simulink model "advanced_3d_lookup"  (R2023a)
settings: Solver=ode1  StartTime=0  StopTime=400  FixedStep=0.002  RelTol=1e-3  EnableMultiTasking=on
values from neighbouring files (symbols this model uses):
  B = b*L*(K_v)^2 /J_xx    (= 0.042375883612)    [advanced_model_setup.m]    (also in brusselator.m = 2.15; cycle_detection.m = img2; cycle_detection_start.m = img2; demonstrateDetections.m = 2.15)
  beta3d = 0.9    [advanced_model_setup.m]
  cycleGain = 0.1    [advanced_model_setup.m]
  epsilon3d = 1    [advanced_model_setup.m]    (also in gainScheduling.m = evalin('base', 'epsilon3d'))
  f_p = 1.3    [advanced_model_setup.m]    (also in modelCompPlot.m)
  f_r = 0.4    [advanced_model_setup.m]    (also in modelCompPlot.m)
  f_y = 0.175    [advanced_model_setup.m]    (also in modelCompPlot.m)
  g_p = 10.5    [advanced_model_setup.m]    (also in modelCompPlot.m)
  g_r = 5.2    [advanced_model_setup.m]    (also in modelCompPlot.m)
  I_xx = 0.0522    [advanced_model_setup.m]    (also in modelCompPlot.m; set_model_params.m; solveSyms3d_2.m = evalin('base', 'I_xx'))
  I_yy = 0.0522    [advanced_model_setup.m]    (also in modelCompPlot.m; set_model_params.m; solveSyms3d_2.m = evalin('base', 'I_yy'))
  I_zz = 0.1104    [advanced_model_setup.m]    (also in modelCompPlot.m; set_model_params.m; solveSyms3d_2.m = evalin('base', 'I_zz'))
  J = (J_yy - J_zz)/J_xx    (= -1)    [advanced_model_setup.m]    (also in modelCompPlot.m)
  J_r = J_inertia/J_xx    (= 0.00108695652174)    [advanced_model_setup.m]    (also in modelCompPlot.m; solveSyms3d.m = evalin('base', 'J_r'))
  k3d = 1.65    [advanced_model_setup.m]    (also in gainScheduling.m = evalin('base', 'k3d'))
  K_v = 54.945    [advanced_model_setup.m]    (also in modelCompPlot.m; solveSyms3d.m = evalin('base', 'K_v'))
  kfr_p = 0.4*u2line/x5line    (= 0.285774113641)    [advanced_model_setup.m]    (also in modelCompPlot.m; set_model_params.m)
  kfr_r = 0.4*u1line/x4line    (= 0.285774113641)    [advanced_model_setup.m]    (also in modelCompPlot.m; set_model_params.m)
  kfr_y = 0.4*u3line/x6line    (= 0.0880063173321)    [advanced_model_setup.m]    (also in modelCompPlot.m; set_model_params.m)
  sigma = 0    [modelCompPlot.m]
  u1_T = zeros(x5L, x6L, u10L, u20L)    [lookup_gen_optimal.m]
  u2_T = zeros(x5L, x6L, u10L, u20L)    [lookup_gen_optimal.m]
  u3_T = zeros(x5L, x6L, u10L, u20L)    [lookup_gen_optimal.m]
  u4_T = zeros(x5L, x6L, u10L, u20L)    [lookup_gen_optimal.m]
  V_bias = 12    [advanced_model_setup.m]    (also in modelCompPlot.m; set_model_params.m; solveSyms3d.m = evalin('base', 'V_bias'))
  velMax = 1000    [advanced_model_setup.m]
  wcf = 2 * pi * 20    (= 125.663706144)    [advanced_model_setup.m]    (also in modelCompPlot.m; set_model_params.m)
  x5_range = -45:5:45    [lookup_gen_optimal.m]
  x6_range = -45:5:45    [lookup_gen_optimal.m]
  Y = d*(K_v)^2 /J_zz    (= 0.0032609614876)    [advanced_model_setup.m]    (also in modelCompPlot.m; solveSyms3d.m = evalin('base', 'Y'))
  zetaf = 0.6    [advanced_model_setup.m]    (also in modelCompPlot.m; set_model_params.m)
undefined symbols (not defined in the file or in its folder): u00_range
libraries: simulink_extras x2, dspsrcs4 x1
settings Model: ExtModeTrigDuration=10000  Creator=kille  LastModifiedBy=Jacob
settings SolverCC: PositivePriorityOrder=on  AutoInsertRateTranBlk=on
settings DataIOCC: ReturnWorkspaceOutputs=off
settings OptimizationCC: LifeSpan=inf
settings DebuggingCC: UnconnectedInputMsg=warning  UnconnectedOutputMsg=warning  UnconnectedLineMsg=warning  ArithmeticOperatorsInVariantConditions=warning
settings ModelReferenceCC: EnableRefExpFcnMdlSchedulingChecks=on
settings SFSimCC: SimUseLocalCustomCode=off  CustomCodeUndefinedFunction=UseInterfaceOnly
settings RTWCC: Description=QUARC Win64 Target  SystemTargetFile=quarc_win64.tlc  TemplateMakefile=quarc_default_tmf  RTWUseLocalCustomCode=off
settings CodeAppCC: StateflowObjectComments=on
settings STFCustomTargetCC: TargetPreCompLibLocation=C:\PROGRA~3\QUARC\lib\2016a\win64\release  UseToolchainInfoCompliant=off  SystemTargetFile=quarc_win64.tlc
settings GRTTargetCC: TargetPreCompLibLocation=C:\PROGRA~3\QUARC\lib\2016a\win64\release  ParMdlRefBuildCompliant=off  CompOptLevelCompliant=off  CombineOutputUpdateFcns=off  MatFileLogging=off  CPPClassGenCompliant=off  GRTInterface=on  UseToolchainInfoCompliant=off  ExtMode=on  ExtModeMexFile=quarc_comm
settings ConfigComp: CovMetricSettings=dswe

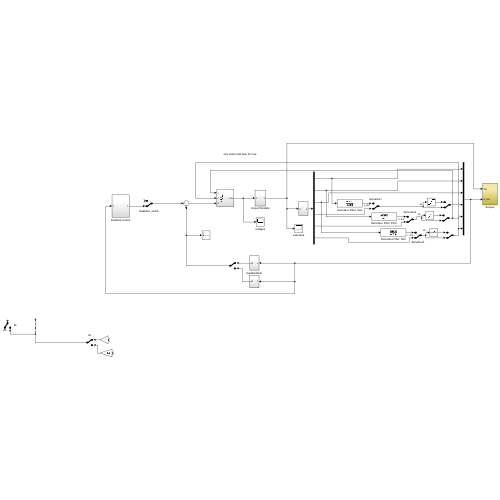
[thumbnail: Simulink's stored preview of the top-level diagram]
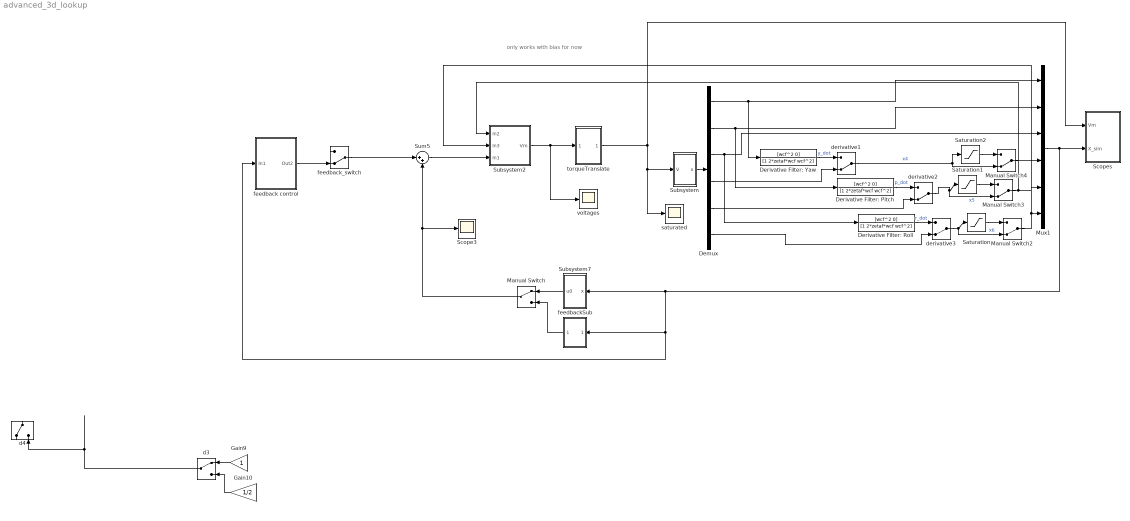
== system advanced_3d_lookup ==
  note: only works with bias for now
  Demux : Demux  Outputs=6
  Derivative Filter: Pitch : TransferFcn  Numerator=[wcf^2 0]  Denominator=[1 2*zetaf*wcf wcf^2]
  Derivative Filter: Roll : TransferFcn  Numerator=[wcf^2 0]  Denominator=[1 2*zetaf*wcf wcf^2]
  Derivative Filter: Yaw : TransferFcn  Numerator=[wcf^2 0]  Denominator=[1 2*zetaf*wcf wcf^2]
  Gain10 : Gain  Gain=1/2
  Gain9 : Gain
  Manual Switch : ManualSwitch
  Manual Switch2 : ManualSwitch  CurrentSetting=0
  Manual Switch3 : ManualSwitch  CurrentSetting=0
  Manual Switch4 : ManualSwitch  CurrentSetting=0
  Mux1 : Mux  Inputs=6
  Saturation : Saturate  UpperLimit=velMax  LowerLimit=-velMax
  Saturation1 : Saturate  UpperLimit=velMax  LowerLimit=-velMax
  Saturation2 : Saturate  UpperLimit=velMax  LowerLimit=-velMax
  Scope3 : Scope
  Scopes : Subsystem
  Subsystem : Subsystem
  Subsystem2 : Subsystem
  Subsystem7 : Subsystem
  Sum5 : Sum  Inputs=|++
  d3 : ManualSwitch
  d4 : ManualSwitch
  derivative1 : ManualSwitch  CurrentSetting=0
  derivative2 : ManualSwitch  CurrentSetting=0
  derivative3 : ManualSwitch  CurrentSetting=0
  feedback control : Subsystem
  feedbackSub : Subsystem
  feedback_switch : ManualSwitch  CurrentSetting=0
  saturated : Scope
  torqueTranslate : Subsystem
  voltages : Scope
  wires:
  Gain10/1 -> d3/2
  d3/1 -> d4/2
  Gain9/1 -> d3/1
  derivative2/1 -> Manual Switch3/2, Saturation1/1  "x5"
  Derivative Filter: Pitch/1 -> derivative2/1  "p_dot"
  Saturation2/1 -> Manual Switch4/1
  Saturation1/1 -> Manual Switch3/1
  Saturation/1 -> Manual Switch2/1
  Demux/4 -> derivative1/2
  derivative1/1 -> Saturation2/1, Manual Switch4/2  "x4"
  derivative3/1 -> Manual Switch2/2, Saturation/1  "x6"
  Derivative Filter: Roll/1 -> derivative3/1  "r_dot"
  Derivative Filter: Yaw/1 -> derivative1/1  "y_dot"
  Subsystem/1(x) -> Demux/1
  Manual Switch4/1 -> Mux1/4
  Manual Switch3/1 -> Subsystem2/1(In2), Mux1/5
  Manual Switch2/1 -> Mux1/6, Subsystem2/2(In3)
  Demux/1 -> Derivative Filter: Yaw/1, Mux1/1
  Demux/2 -> Derivative Filter: Pitch/1, Mux1/2
  Demux/3 -> Derivative Filter: Roll/1, Mux1/3
  Demux/5 -> derivative2/2
  Demux/6 -> derivative3/2
  Mux1/1 -> feedbackSub/1(Input), feedback control/1(In1), Subsystem7/1(x), Scopes/2(X_sim)
  Subsystem2/1(Vm) -> torqueTranslate/1(In1), voltages/1
  Sum5/1 -> Subsystem2/3(In1)
  feedback control/1(Out2) -> feedback_switch/2
  feedback_switch/1 -> Sum5/1
  Subsystem7/1(u0) -> Manual Switch/1
  feedbackSub/1(u0) -> Manual Switch/2
  Manual Switch/1 -> Sum5/2, Scope3/1
  torqueTranslate/1(Out1) -> Scopes/1(Vm), saturated/1, Subsystem/1(V)

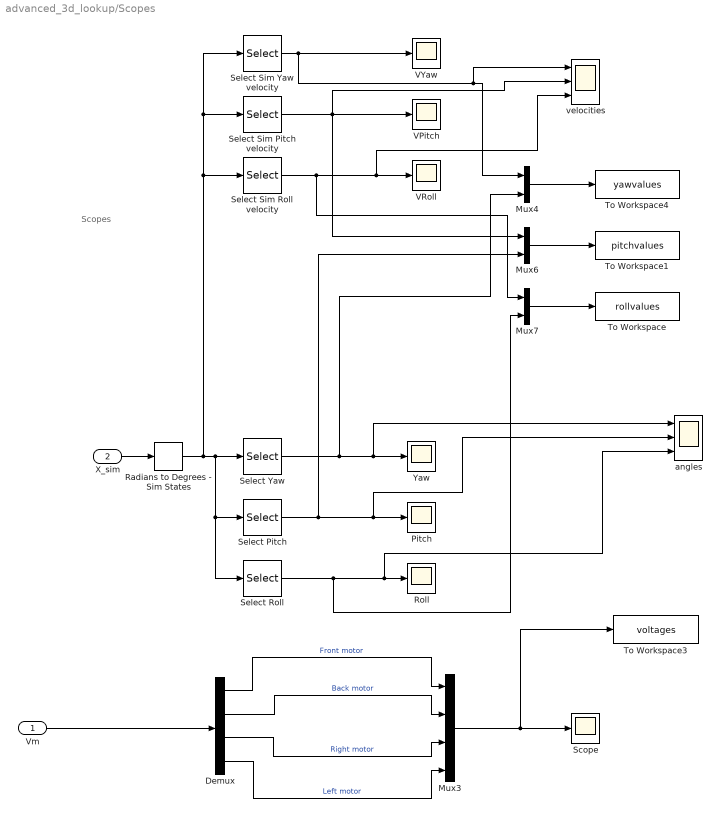
== system advanced_3d_lookup/Scopes ==
  note: Scopes
  Vm : Inport
  X_sim : Inport  Port=2
  Demux : Demux
  Mux3 : Mux
  Mux4 : Mux  Inputs=2
  Mux6 : Mux  Inputs=2
  Mux7 : Mux  Inputs=2
  Pitch : Scope
  Radians to Degrees - Sim States : simulink_extras/Transformations/Radians to Degrees
  Roll : Scope
  Scope : Scope
  Select Pitch : Selector  InputPortWidth=6  IndexOptions=Index vector (dialog)  Indices=2  OutputSizes=1
  Select Roll : Selector  InputPortWidth=6  IndexOptions=Index vector (dialog)  Indices=3  OutputSizes=1
  Select Sim Pitch velocity : Selector  InputPortWidth=6  IndexOptions=Index vector (dialog)  Indices=5  OutputSizes=1
  Select Sim Roll velocity : Selector  InputPortWidth=6  IndexOptions=Index vector (dialog)  Indices=6  OutputSizes=1
  Select Sim Yaw velocity : Selector  InputPortWidth=6  IndexOptions=Index vector (dialog)  Indices=4  OutputSizes=1
  Select Yaw : Selector  InputPortWidth=6  IndexOptions=Index vector (dialog)  Indices=1  OutputSizes=1
  To Workspace : ToWorkspace  VariableName=rollvalues  SampleTime=-1
  To Workspace1 : ToWorkspace  VariableName=pitchvalues  SampleTime=-1
  To Workspace3 : ToWorkspace  VariableName=voltages  SampleTime=-1
  To Workspace4 : ToWorkspace  VariableName=yawvalues  SampleTime=-1
  VPitch : Scope
  VRoll : Scope
  VYaw : Scope
  Yaw : Scope
  angles : Scope  NumInputPorts=3
  velocities : Scope  NumInputPorts=3
  wires:
  Select Roll/1 -> angles/3, Roll/1, Mux7/2
  Radians to Degrees - Sim States/1 -> Select Sim Roll velocity/1, Select Sim Pitch velocity/1, Select Sim Yaw velocity/1, Select Roll/1, Select Pitch/1, Select Yaw/1
  Select Pitch/1 -> angles/2, Pitch/1, Mux6/2
  X_sim/1 -> Radians to Degrees - Sim States/1
  Demux/1 -> Mux3/1  "Front motor"
  Demux/2 -> Mux3/2  "Back motor"
  Demux/3 -> Mux3/3  "Right motor"
  Demux/4 -> Mux3/4  "Left motor"
  Vm/1 -> Demux/1
  Select Sim Yaw velocity/1 -> VYaw/1, velocities/1, Mux4/1
  Select Sim Roll velocity/1 -> velocities/3, VRoll/1, Mux7/1
  Select Sim Pitch velocity/1 -> Mux6/1, velocities/2, VPitch/1
  Mux4/1 -> To Workspace4/1
  Mux6/1 -> To Workspace1/1
  Mux7/1 -> To Workspace/1
  Mux3/1 -> To Workspace3/1, Scope/1
  Select Yaw/1 -> angles/1, Yaw/1, Mux4/2

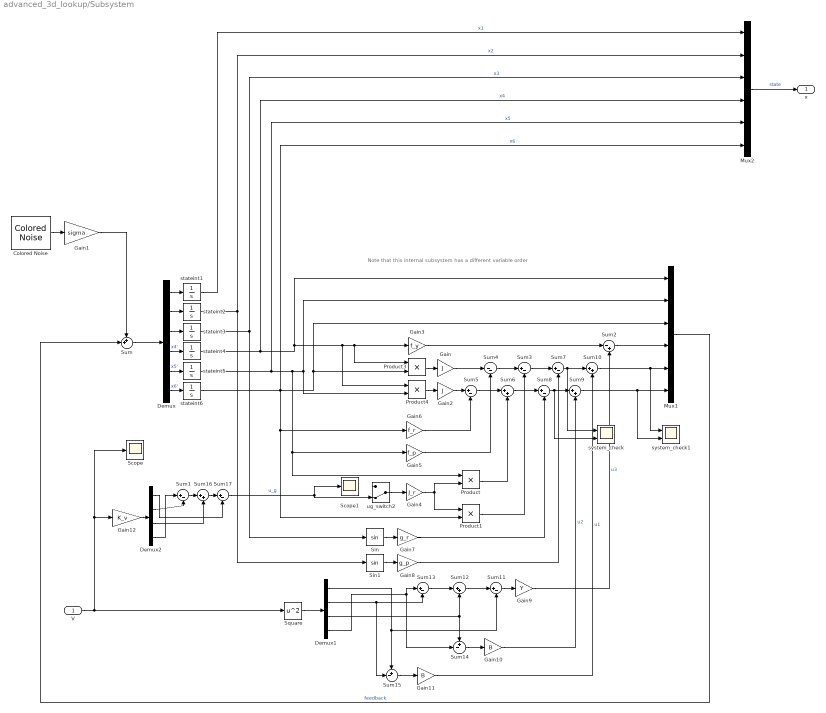
== system advanced_3d_lookup/Subsystem ==
  note: Note that this internal subsystem has a different variable order
  V : Inport
  Colored Noise : dspsrcs4/Colored Noise  Color=white  InverseFrequencyPower=1  BoundedOutput=off  NumChannels=6  OutputDataType=double  SamplesPerFrame=1  SampleTime=1  RandomStream=mt19937ar with seed  Seed=67  SimulateUsing=Interpreted execution
  Demux : Demux  Outputs=6
  Demux1 : Demux
  Demux2 : Demux
  Gain : Gain  Gain=J
  Gain1 : Gain  Gain=sigma
  Gain10 : Gain  Gain=B
  Gain11 : Gain  Gain=B
  Gain12 : Gain  Gain=K_v
  Gain2 : Gain  Gain=J
  Gain3 : Gain  Gain=f_y
  Gain4 : Gain  Gain=J_r
  Gain5 : Gain  Gain=f_p
  Gain6 : Gain  Gain=f_r
  Gain7 : Gain  Gain=g_r
  Gain8 : Gain  Gain=g_p
  Gain9 : Gain  Gain=Y
  Mux1 : Mux  Inputs=6
  Mux2 : Mux  Inputs=6
  Product{,1,3..4} (4 alike) : Product
  Scope : Scope
  Scope1 : Scope
  Sin : Trigonometry
  Sin1 : Trigonometry
  Square : Math  Operator=square
  Sum : Sum  Inputs=++|
  Sum{1,3,5,7..8,11,13,17} (8 alike) : Sum  Inputs=|+-
  Sum{6,9..10,12,16} (5 alike) : Sum  Inputs=|++
  Sum14 : Sum  Inputs=+-|
  Sum15 : Sum  Inputs=+-|
  Sum2 : Sum  Inputs=|-+
  Sum4 : Sum  Inputs=|--
  stateint1 : Integrator  InitialCondition=0.017453
  stateint2 : Integrator  InitialCondition=0.017453
  stateint3 : Integrator  InitialCondition=0.017453
  stateint4 : Integrator
  stateint5 : Integrator
  stateint6 : Integrator
  system_check : Scope  NumInputPorts=2
  system_check1 : Scope  NumInputPorts=2
  ug_switch2 : ManualSwitch  CurrentSetting=0
  x : Outport
  wires:
  stateint5/1 -> Mux2/5, Gain5/1, Product/1, Product4/2, Mux1/2  "x5"
  stateint4/1 -> Mux2/4, Mux1/1, Product4/1, Product3/1, Gain3/1  "x4"
  Demux/1 -> stateint1/1
  stateint6/1 -> Mux2/6, Gain6/1, Product1/2, Product3/2, Mux1/3  "x6"
  Demux/6 -> stateint6/1  "x6'"
  Demux/5 -> stateint5/1  "x5'"
  Demux/2 -> stateint2/1
  Demux/3 -> stateint3/1
  Demux/4 -> stateint4/1  "x4'"
  Product3/1 -> Gain/1
  Product4/1 -> Gain2/1
  Colored Noise/1 -> Gain1/1
  Sum/1 -> Demux/1
  Gain1/1 -> Sum/1
  Gain3/1 -> Sum2/1
  Gain4/1 -> Product1/1, Product/2
  Sum17/1 -> ug_switch2/2, Scope1/1  "u_g"
  Gain/1 -> Sum4/1
  Gain2/1 -> Sum5/1
  Gain6/1 -> Sum5/2
  Gain5/1 -> Sum4/2
  Sum5/1 -> Sum6/1
  Product/1 -> Sum6/2
  Sum4/1 -> Sum3/1
  Sum6/1 -> Sum8/1
  Sum3/1 -> Sum7/1
  Gain7/1 -> Sum8/2
  Gain8/1 -> Sum7/2
  Sin/1 -> Gain7/1
  Sin1/1 -> Gain8/1
  Sum8/1 -> system_check/2, Sum9/1
  Sum7/1 -> system_check/1, Sum10/1
  Sum11/1 -> Gain9/1
  Gain9/1 -> Sum2/2  "u3"
  Square/1 -> Demux1/1
  Sum12/1 -> Sum11/1
  Sum13/1 -> Sum12/1
  Demux1/4 -> Sum13/1, Sum14/2
  Demux1/2 -> Sum13/2, Sum15/2
  Demux1/3 -> Sum12/2, Sum14/1
  Demux1/1 -> Sum15/1, Sum11/2
  Sum14/1 -> Gain10/1
  Sum15/1 -> Gain11/1
  Gain10/1 -> Sum9/2  "u2"
  Gain11/1 -> Sum10/2  "u1"
  Mux1/1 -> Sum/2  "feedback"
  V/1 -> Square/1, Scope/1, Gain12/1
  Gain12/1 -> Demux2/1
  Sum1/1 -> Sum16/1
  Sum16/1 -> Sum17/1
  Demux2/2 -> Sum1/2
  Demux2/3 -> Sum16/2
  Sum10/1 -> system_check1/1, Mux1/5
  Sum2/1 -> Mux1/4
  stateint2/1 -> Mux2/2, Sin1/1  "x2"
  stateint3/1 -> Mux2/3, Sin/1  "x3"
  Product1/1 -> Sum3/2
  Demux2/4 -> Sum1/1
  Demux2/1 -> Sum17/2
  stateint1/1 -> Mux2/1  "x1"
  Mux2/1 -> x/1  "state"
  Sum9/1 -> system_check1/2, Mux1/6
  ug_switch2/1 -> Gain4/1

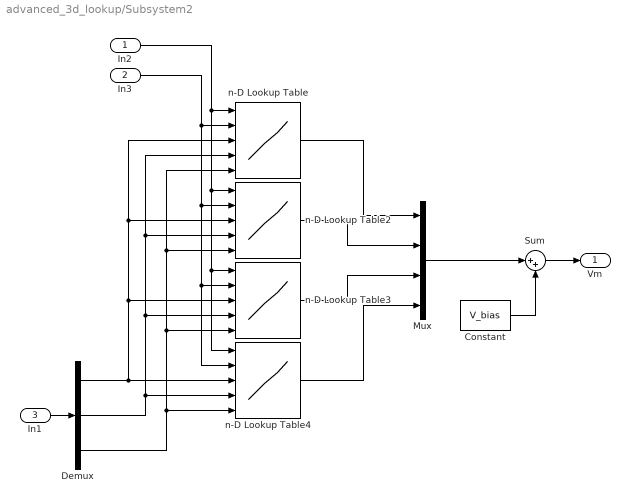
== system advanced_3d_lookup/Subsystem2 ==
  In2 : Inport
  In3 : Inport  Port=2
  In1 : Inport  Port=3
  Constant : Constant  Value=V_bias
  Demux : Demux  Outputs=3
  Mux : Mux
  Sum : Sum  Inputs=|++
  n-D Lookup Table : Lookup_n-D  NumberOfTableDimensions=5  BreakpointsForDimension1=x5_range  BreakpointsForDimension2=x6_range  BreakpointsForDimension3=u00_range  BreakpointsForDimension4=u10_range  BreakpointsForDimension5=u20_range  Table=u1_T  InternalRulePriority=Speed  RndMeth=Simplest
      settings: InputPortMap=u0,u1,u2,u3,u4
  n-D Lookup Table2 : Lookup_n-D  NumberOfTableDimensions=5  BreakpointsForDimension1=x5_range  BreakpointsForDimension2=x6_range  BreakpointsForDimension3=u00_range  BreakpointsForDimension4=u10_range  BreakpointsForDimension5=u20_range  Table=u2_T  InternalRulePriority=Speed  RndMeth=Simplest
      settings: InputPortMap=u0,u1,u2,u3,u4
  n-D Lookup Table3 : Lookup_n-D  NumberOfTableDimensions=5  BreakpointsForDimension1=x5_range  BreakpointsForDimension2=x6_range  BreakpointsForDimension3=u00_range  BreakpointsForDimension4=u10_range  BreakpointsForDimension5=u20_range  Table=u3_T  InternalRulePriority=Speed  RndMeth=Simplest
      settings: InputPortMap=u0,u1,u2,u3,u4
  n-D Lookup Table4 : Lookup_n-D  NumberOfTableDimensions=5  BreakpointsForDimension1=x5_range  BreakpointsForDimension2=x6_range  BreakpointsForDimension3=u00_range  BreakpointsForDimension4=u10_range  BreakpointsForDimension5=u20_range  Table=u4_T  InternalRulePriority=Speed  RndMeth=Simplest
      settings: InputPortMap=u0,u1,u2,u3,u4
  Vm : Outport
  wires:
  In3/1 -> n-D Lookup Table4/2, n-D Lookup Table3/2, n-D Lookup Table2/2, n-D Lookup Table/2
  In2/1 -> n-D Lookup Table2/1, n-D Lookup Table4/1, n-D Lookup Table3/1, n-D Lookup Table/1
  Sum/1 -> Vm/1
  Mux/1 -> Sum/1
  Constant/1 -> Sum/2
  In1/1 -> Demux/1
  Demux/1 -> n-D Lookup Table4/3, n-D Lookup Table3/3, n-D Lookup Table2/3, n-D Lookup Table/3
  Demux/2 -> n-D Lookup Table4/4, n-D Lookup Table3/4, n-D Lookup Table2/4, n-D Lookup Table/4
  Demux/3 -> n-D Lookup Table4/5, n-D Lookup Table3/5, n-D Lookup Table2/5, n-D Lookup Table/5
  n-D Lookup Table/1 -> Mux/1
  n-D Lookup Table2/1 -> Mux/2
  n-D Lookup Table3/1 -> Mux/3
  n-D Lookup Table4/1 -> Mux/4

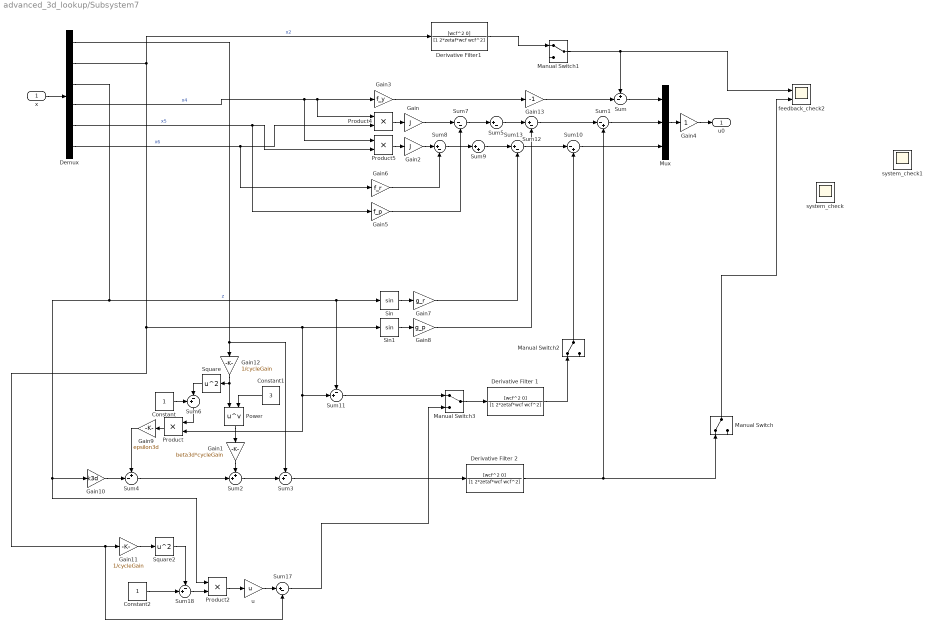
== system advanced_3d_lookup/Subsystem7 ==
  x : Inport
  Constant : Constant
  Constant1 : Constant  Value=3
  Constant2 : Constant
  Demux : Demux  Outputs=6
  Derivative Filter 1 : TransferFcn  Numerator=[wcf^2 0]  Denominator=[1 2*zetaf*wcf wcf^2]
  Derivative Filter 2 : TransferFcn  Numerator=[wcf^2 0]  Denominator=[1 2*zetaf*wcf wcf^2]
  Derivative Filter1 : TransferFcn  Numerator=[wcf^2 0]  Denominator=[1 2*zetaf*wcf wcf^2]
  Gain : Gain  Gain=J
  Gain1 : Gain  Gain=beta3d*cycleGain
  Gain10 : Gain  Gain=k3d
  Gain11 : Gain  Gain=1/cycleGain
  Gain12 : Gain  Gain=1/cycleGain
  Gain13 : Gain  Gain=-1
  Gain2 : Gain  Gain=J
  Gain3 : Gain  Gain=f_y
  Gain4 : Gain
  Gain5 : Gain  Gain=f_p
  Gain6 : Gain  Gain=f_r
  Gain7 : Gain  Gain=g_r
  Gain8 : Gain  Gain=g_p
  Gain9 : Gain  Gain=epsilon3d
  Manual Switch{,1..3} (4 alike) : ManualSwitch
  Mux : Mux  Inputs=3
  Power : Math  Operator=pow
  Product{,2,4..5} (4 alike) : Product
  Sin : Trigonometry
  Sin1 : Trigonometry
  Square : Math  Operator=square
  Square2 : Math  Operator=square
  Sum : Sum  Inputs=+-|
  Sum1 : Sum  Inputs=|-+
  Sum10 : Sum  Inputs=|-+
  Sum11 : Sum  Inputs=-+|
  Sum{5,8,12..13,17} (5 alike) : Sum  Inputs=|+-
  Sum18 : Sum  Inputs=-+|
  Sum2 : Sum  Inputs=++|
  Sum3 : Sum  Inputs=-+|
  Sum4 : Sum  Inputs=+-|
  Sum6 : Sum  Inputs=+-|
  Sum7 : Sum  Inputs=|--
  Sum9 : Sum  Inputs=|++
  feedback_check2 : Scope  NumInputPorts=2
  system_check : Scope  NumInputPorts=2
  system_check1 : Scope  NumInputPorts=2
  u : Gain  Gain=u
  u0 : Outport
  wires:
  Derivative Filter 2/1 -> Manual Switch/1, Sum1/2
  Derivative Filter1/1 -> Manual Switch1/1
  Manual Switch/1 -> feedback_check2/2
  Manual Switch1/1 -> feedback_check2/1, Sum/1
  x/1 -> Demux/1
  Demux/5 -> Gain5/1, Product5/2  "x5"
  Sin/1 -> Gain7/1
  Product4/1 -> Gain/1
  Gain7/1 -> Sum13/2
  Product5/1 -> Gain2/1
  Sum7/1 -> Sum5/1
  Gain6/1 -> Sum8/2
  Sum8/1 -> Sum9/1
  Gain5/1 -> Sum7/2
  Gain/1 -> Sum7/1
  Sum5/1 -> Sum12/1
  Sum9/1 -> Sum13/1
  Sin1/1 -> Gain8/1
  Gain8/1 -> Sum12/2
  Demux/4 -> Product5/1, Product4/1, Gain3/1  "x4"
  Demux/3 -> Product2/1, Gain10/1, Sin/1, Sum11/1  "z"
  Demux/6 -> Gain6/1, Product4/2  "x6"
  Gain2/1 -> Sum8/1
  Mux/1 -> Gain4/1
  Gain4/1 -> u0/1
  Gain3/1 -> Gain13/1
  Demux/1 -> Sum3/1, Gain12/1
  Product/1 -> Gain9/1
  Square/1 -> Sum6/2
  Gain10/1 -> Sum4/2
  Sum4/1 -> Sum2/2
  Constant/1 -> Sum6/1
  Gain1/1 -> Sum2/1
  Power/1 -> Gain1/1
  Gain9/1 -> Sum4/1
  Sum6/1 -> Product/1
  Sum2/1 -> Sum3/2
  Constant1/1 -> Power/2
  Sum3/1 -> Derivative Filter 2/1
  Sum12/1 -> Sum1/1
  Sum13/1 -> Sum10/1
  Sum10/1 -> Mux/3
  Constant2/1 -> Sum18/2
  Sum18/1 -> Product2/2
  Gain11/1 -> Square2/1
  u/1 -> Sum17/1
  Square2/1 -> Sum18/1
  Product2/1 -> u/1
  Demux/2 -> Sum17/2, Gain11/1, Sum11/2, Product/2, Sin1/1, Derivative Filter1/1  "x2"
  Manual Switch3/1 -> Derivative Filter 1/1
  Sum11/1 -> Manual Switch3/1
  Sum17/1 -> Manual Switch3/2
  Sum1/1 -> Mux/2
  Gain12/1 -> Square/1, Power/1
  Gain13/1 -> Sum/2
  Sum/1 -> Mux/1
  Derivative Filter 1/1 -> Manual Switch2/1
  Manual Switch2/1 -> Sum10/2

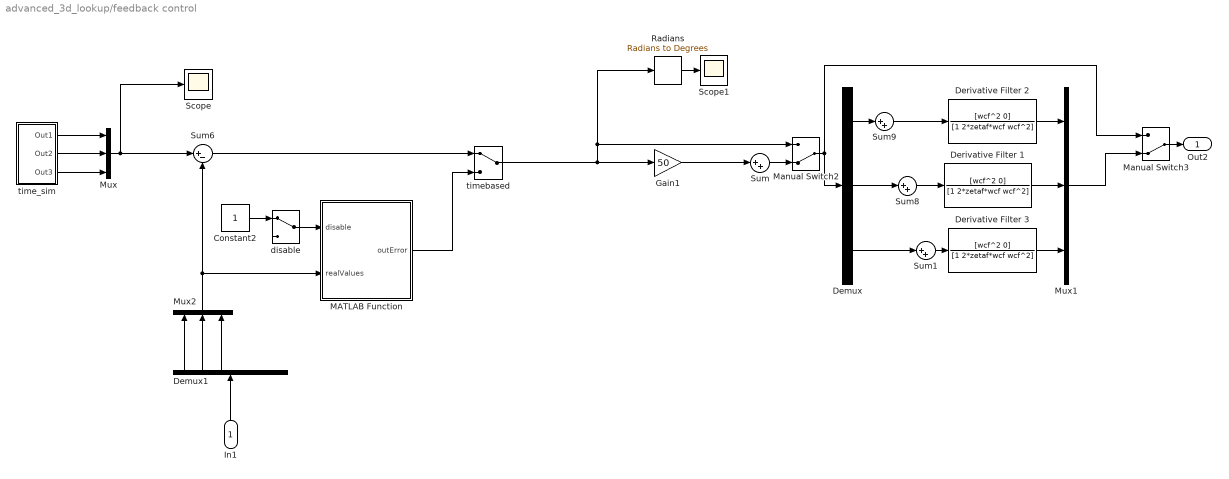
== system advanced_3d_lookup/feedback control ==
  In1 : Inport
  Constant2 : Constant
  Demux : Demux  Outputs=3
  Demux1 : Demux  Outputs=6
  Derivative Filter 1 : TransferFcn  Numerator=[wcf^2 0]  Denominator=[1 2*zetaf*wcf wcf^2]
  Derivative Filter 2 : TransferFcn  Numerator=[wcf^2 0]  Denominator=[1 2*zetaf*wcf wcf^2]
  Derivative Filter 3 : TransferFcn  Numerator=[wcf^2 0]  Denominator=[1 2*zetaf*wcf wcf^2]
  Gain1 : Gain  Gain=50
  MATLAB Function : MATLAB Function  TreatAsAtomicUnit=on
  Manual Switch2 : ManualSwitch  CurrentSetting=0
  Manual Switch3 : ManualSwitch  CurrentSetting=0
  Mux : Mux  Inputs=3
  Mux1 : Mux  Inputs=3
  Mux2 : Mux  Inputs=3
  Radians : simulink_extras/Transformations/Radians to Degrees
  Scope : Scope
  Scope1 : Scope
  Sum{,1,8..9} (4 alike) : Sum  Inputs=|++
  Sum6 : Sum  Inputs=|+-
  disable : ManualSwitch
  time_sim : Subsystem
  timebased : ManualSwitch
  Out2 : Outport
  wires:
  Mux/1 -> Scope/1, Sum6/1
  Demux1/2 -> Mux2/2
  Demux1/1 -> Mux2/1
  Demux1/3 -> Mux2/3
  In1/1 -> Demux1/1
  MATLAB Function/1(outError) -> timebased/2
  Sum6/1 -> timebased/1
  Mux2/1 -> MATLAB Function/2(realValues), Sum6/2
  Constant2/1 -> disable/1
  time_sim/1(Out1) -> Mux/1
  time_sim/2(Out2) -> Mux/2
  time_sim/3(Out3) -> Mux/3
  Demux/1 -> Sum9/1
  Demux/2 -> Sum8/1
  timebased/1 -> Manual Switch2/1, Radians/1, Gain1/1
  Derivative Filter 1/1 -> Mux1/2
  Manual Switch3/1 -> Out2/1
  Radians/1 -> Scope1/1
  Sum/1 -> Manual Switch2/2
  Gain1/1 -> Sum/1
  Manual Switch2/1 -> Manual Switch3/1, Demux/1
  Derivative Filter 2/1 -> Mux1/1
  Sum8/1 -> Derivative Filter 1/1
  Mux1/1 -> Manual Switch3/2
  Sum9/1 -> Derivative Filter 2/1
  Sum1/1 -> Derivative Filter 3/1
  Derivative Filter 3/1 -> Mux1/3
  Demux/3 -> Sum1/1
  disable/1 -> MATLAB Function/1(disable)

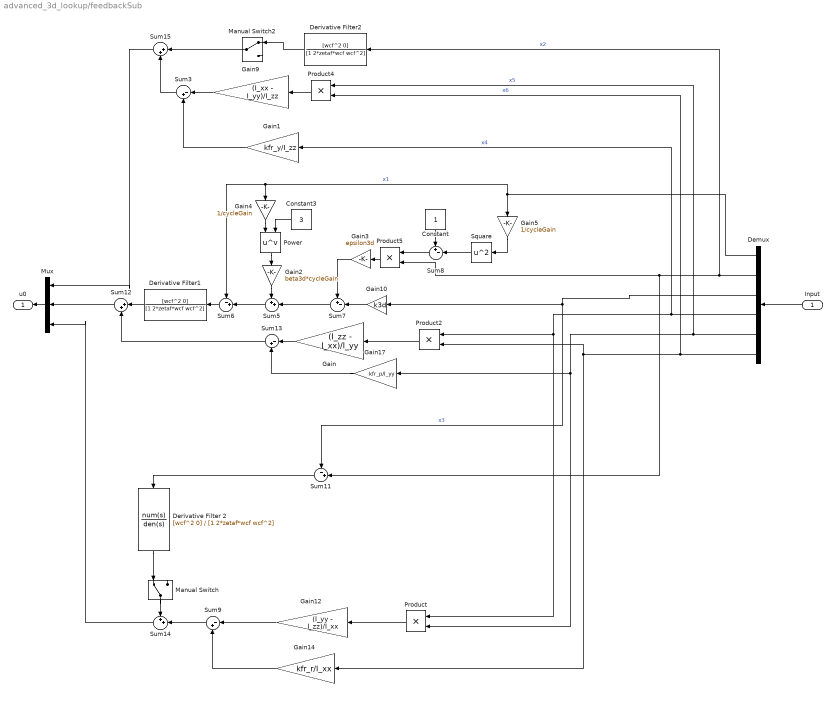
== system advanced_3d_lookup/feedbackSub ==
  Input : Inport
  Constant : Constant
  Constant3 : Constant  Value=3
  Demux : Demux  Outputs=6
  Derivative Filter 2 : TransferFcn  Numerator=[wcf^2 0]  Denominator=[1 2*zetaf*wcf wcf^2]
  Derivative Filter1 : TransferFcn  Numerator=[wcf^2 0]  Denominator=[1 2*zetaf*wcf wcf^2]
  Derivative Filter2 : TransferFcn  Numerator=[wcf^2 0]  Denominator=[1 2*zetaf*wcf wcf^2]
  Gain : Gain  Gain=(I_zz - I_xx)/I_yy
  Gain1 : Gain  Gain=kfr_y/I_zz
  Gain10 : Gain  Gain=k3d
  Gain12 : Gain  Gain=(I_yy - I_zz)/I_xx
  Gain14 : Gain  Gain=kfr_r/I_xx
  Gain17 : Gain  Gain=kfr_p/I_yy
  Gain2 : Gain  Gain=beta3d*cycleGain
  Gain3 : Gain  Gain=epsilon3d
  Gain4 : Gain  Gain=1/cycleGain
  Gain5 : Gain  Gain=1/cycleGain
  Gain9 : Gain  Gain=(I_xx - I_yy)/I_zz
  Manual Switch : ManualSwitch
  Manual Switch2 : ManualSwitch
  Mux : Mux  Inputs=3
  Power : Math  Operator=pow
  Product{,2,4..5} (4 alike) : Product
  Square : Math  Operator=square
  Sum11 : Sum  Inputs=-+|
  Sum12 : Sum  Inputs=|++
  Sum13 : Sum  Inputs=|-+
  Sum14 : Sum  Inputs=++|
  Sum15 : Sum  Inputs=|++
  Sum3 : Sum  Inputs=|-+
  Sum5 : Sum  Inputs=++|
  Sum6 : Sum  Inputs=-+|
  Sum7 : Sum  Inputs=+-|
  Sum8 : Sum  Inputs=+-|
  Sum9 : Sum  Inputs=|-+
  u0 : Outport
  wires:
  Gain17/1 -> Sum13/2
  Sum13/1 -> Sum12/2
  Demux/4 -> Product/1, Product2/1, Gain1/1  "x4"
  Product2/1 -> Gain/1
  Demux/5 -> Product4/1, Product/2, Gain17/1  "x5"
  Product/1 -> Gain12/1
  Demux/6 -> Gain14/1, Product2/2, Product4/2  "x6"
  Manual Switch/1 -> Sum14/1
  Sum9/1 -> Sum14/2
  Gain12/1 -> Sum9/1
  Gain/1 -> Sum13/1
  Gain14/1 -> Sum9/2
  Sum12/1 -> Mux/2
  Derivative Filter 2/1 -> Manual Switch/1
  Sum14/1 -> Mux/3
  Input/1 -> Demux/1
  Demux/3 -> Gain10/1, Sum11/1  "x3"
  Product4/1 -> Gain9/1
  Gain9/1 -> Sum3/1
  Gain1/1 -> Sum3/2
  Gain3/1 -> Sum7/1
  Gain2/1 -> Sum5/1
  Constant/1 -> Sum8/1
  Constant3/1 -> Power/2
  Square/1 -> Sum8/2
  Sum8/1 -> Product5/1
  Gain10/1 -> Sum7/2
  Sum7/1 -> Sum5/2
  Sum5/1 -> Sum6/2
  Product5/1 -> Gain3/1
  Power/1 -> Gain2/1
  Manual Switch2/1 -> Sum15/1
  Demux/2 -> Derivative Filter2/1, Product5/2, Sum11/2  "x2"
  Derivative Filter2/1 -> Manual Switch2/1
  Sum3/1 -> Sum15/2
  Demux/1 -> Gain4/1, Sum6/1, Gain5/1  "x1"
  Derivative Filter1/1 -> Sum12/1
  Sum6/1 -> Derivative Filter1/1
  Sum11/1 -> Derivative Filter 2/1
  Sum15/1 -> Mux/1
  Mux/1 -> u0/1
  Gain4/1 -> Power/1
  Gain5/1 -> Square/1

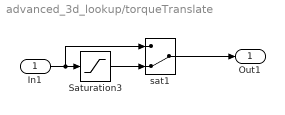
== system advanced_3d_lookup/torqueTranslate ==
  In1 : Inport
  Saturation3 : Saturate  UpperLimit=24  LowerLimit=-24
  sat1 : ManualSwitch  CurrentSetting=0
  Out1 : Outport
  wires:
  In1/1 -> sat1/1, Saturation3/1
  Saturation3/1 -> sat1/2
  sat1/1 -> Out1/1

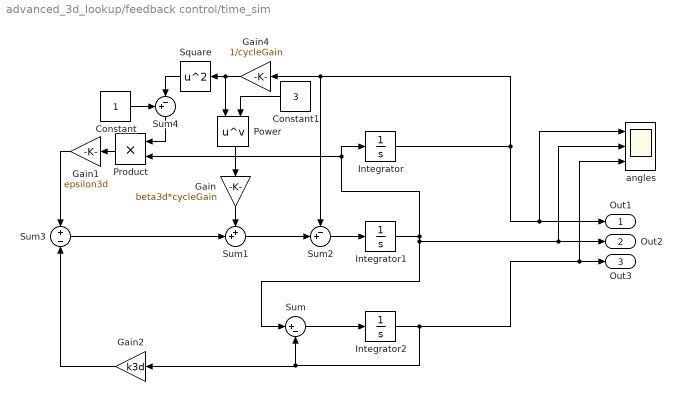
== system advanced_3d_lookup/feedback control/time_sim ==
  Constant : Constant
  Constant1 : Constant  Value=3
  Gain : Gain  Gain=beta3d*cycleGain
  Gain1 : Gain  Gain=epsilon3d
  Gain2 : Gain  Gain=k3d
  Gain4 : Gain  Gain=1/cycleGain
  Integrator : Integrator  InitialCondition=0.0001
  Integrator1 : Integrator  InitialCondition=0.0001
  Integrator2 : Integrator  InitialCondition=0.0001
  Power : Math  Operator=pow
  Product : Product
  Square : Math  Operator=square
  Sum : Sum  Inputs=|+-
  Sum1 : Sum  Inputs=++|
  Sum2 : Sum  Inputs=-+|
  Sum3 : Sum  Inputs=+|-
  Sum4 : Sum  Inputs=+-|
  angles : Scope  NumInputPorts=3
  Out1 : Outport
  Out2 : Outport  Port=2
  Out3 : Outport  Port=3
  wires:
  Gain4/1 -> Square/1, Power/1
  Product/1 -> Gain1/1
  Constant/1 -> Sum4/1
  Sum3/1 -> Sum1/2
  Sum2/1 -> Integrator1/1
  Gain/1 -> Sum1/1
  Gain2/1 -> Sum3/2
  Square/1 -> Sum4/2
  Sum1/1 -> Sum2/2
  Power/1 -> Gain/1
  Gain1/1 -> Sum3/1
  Constant1/1 -> Power/2
  Sum/1 -> Integrator2/1
  Integrator2/1 -> angles/3, Out3/1, Sum/2, Gain2/1
  Sum4/1 -> Product/1
  Integrator1/1 -> angles/2, Out2/1, Sum/1, Product/2, Integrator/1
  Integrator/1 -> Out1/1, angles/1, Gain4/1, Sum2/1

== matlab function advanced_3d_lookup/feedback control/MATLAB Function ==
  data: disable input; realValues input; outError output
function outError = approxLimitSimu(disable, realValues)
    outError = [0; 0; 0];
    cyclePoint = [0; 0; 0];
    coder.extrinsic('approxLimit');
    if disable ~= 1
        cyclePoint = approxLimit(realValues);
        outError = cyclePoint - realValues;
    end
